simulink model "Electromech_sys_current_lin_obs"  (R2025b)
settings: Solver=VariableStepAuto  StartTime=0.0  StopTime=10.0  RelTol=1e-3
values from neighbouring files (symbols this model uses):
  A = (J - R) * Hxx    [linearize_electromech.m]    (also in linearize_mech.m = (J - R) * Hxx + grad_g * u_eq_mech)
  B = g    [linearize_electromech.m]    (also in linearize_mech.m)
  i_eq = - (1/re) * dHdQ_eq + (1/re) * u_op    [equilibrium_electromech.m]
  p_0 = 0    [Init_Simulink_param_lin_Electromech.m]
  ptilde_0 = phat_0 - x_eq(2)    [Init_Simulink_param_lin_Electromech.m]
  q_0 = 0    [Init_Simulink_param_lin_Electromech.m]
  Q_0 = 0    [Init_Simulink_param_lin_Electromech.m]
  qtilde_0 = qhat_0 - x_eq(1)    [Init_Simulink_param_lin_Electromech.m]
  Qtilde_0 = Qhat_0 - x_eq(3)    [Init_Simulink_param_lin_Electromech.m]
  x_eq = [q_eq; p_eq; Q_eq]    [equilibrium_electromech.m]
undefined symbols (not defined in the file or in its folder): Cnum, params, u_eq
settings Model: Creator=filippougolini  LastModifiedBy=filippougolini

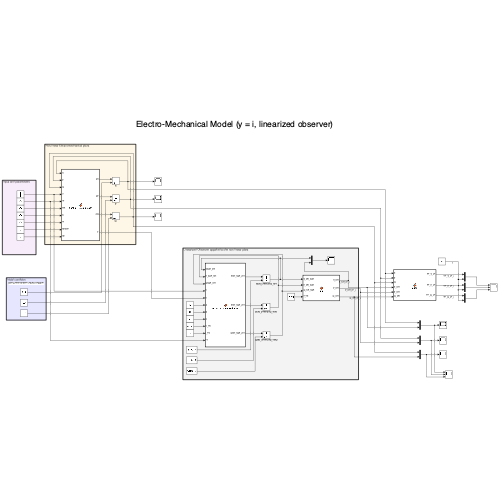
[thumbnail: Simulink's stored preview of the top-level diagram]
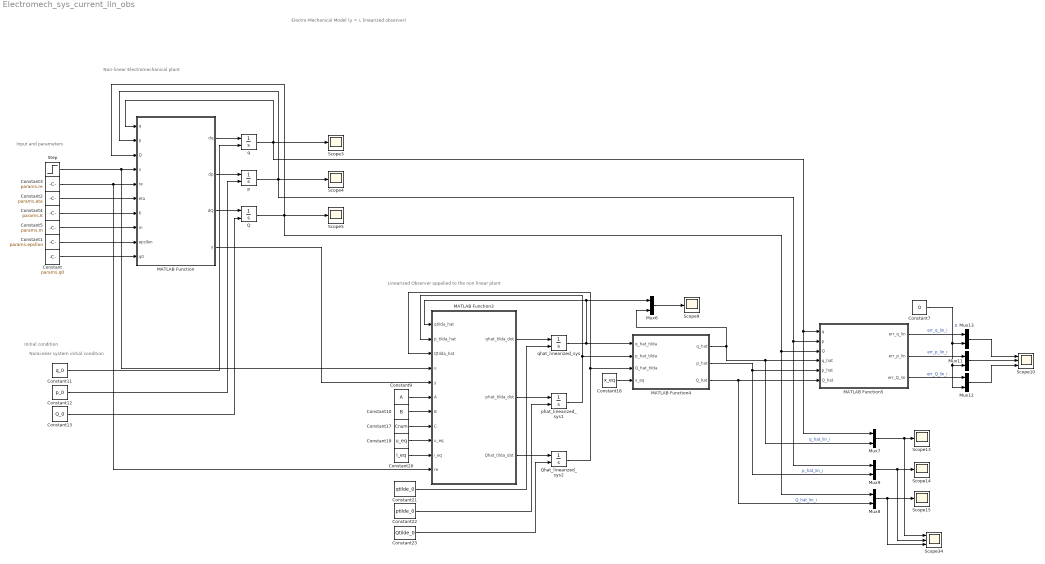
== system Electromech_sys_current_lin_obs ==
  note: Linearized Observer appalied to the non linear plant
  note: Input and parameters
  note: NonLinear system initial condition
  note: Non-linear Electromechanical plant
  note: Electro-Mechanical Model (y = i, linearized observer)
  note: Initial condition
  Constant : Constant  Value=params.q0
  Constant1 : Constant  Value=params.epsllon
  Constant10 : Constant  Value=B
  Constant11 : Constant  Value=q_0
  Constant12 : Constant  Value=p_0
  Constant13 : Constant  Value=Q_0
  Constant17 : Constant  Value=Cnum
  Constant18 : Constant  Value=x_eq
  Constant19 : Constant  Value=u_eq
  Constant2 : Constant  Value=params.eta
  Constant20 : Constant  Value=i_eq
  Constant21 : Constant  Value=qtilde_0
  Constant22 : Constant  Value=ptilde_0
  Constant23 : Constant  Value=Qtilde_0
  Constant3 : Constant  Value=params.re
  Constant4 : Constant  Value=params.K
  Constant5 : Constant  Value=params.m
  Constant7 : Constant  Value=0
  Constant9 : Constant  Value=A
  MATLAB Function : MATLAB Function  TreatAsAtomicUnit=on
  MATLAB Function3 : MATLAB Function  TreatAsAtomicUnit=on
  MATLAB Function4 : MATLAB Function  TreatAsAtomicUnit=on
  MATLAB Function5 : MATLAB Function  TreatAsAtomicUnit=on
  Mux{6..9,11..13} (7 alike) : Mux  Inputs=2
  Q : Integrator  InitialConditionSource=external
  Qhat_linearized_sys2 : Integrator  InitialConditionSource=external  InitialCondition=20e-5
  Scope10 : Scope  NumInputPorts=3
      settings: ActiveDisplayString=3  ActiveDisplayYMinimum=-9.7438576334412446E-8  ActiveDisplayYMaximum=3.7694718700971209E-7  DataLoggingVariableName=ScopeData10
  Scope{3..5,9,13..15} (7 alike) : Scope
      Scope13 settings: ActiveDisplayYMinimum=-0.00014562196235781276  ActiveDisplayYMaximum=0.0013105976612203152  DataLoggingVariableName=ScopeData13
      Scope14 settings: ActiveDisplayYMinimum=-0.0045902088543352884  ActiveDisplayYMaximum=0.00516486271210546  DataLoggingVariableName=ScopeData14
      Scope15 settings: ActiveDisplayYMinimum=-2.096197823231283E-8  ActiveDisplayYMaximum=1.8865780409081551E-7  DataLoggingVariableName=ScopeData15
      Scope3 settings: ActiveDisplayYMinimum=-4.0944874698701246E-5  ActiveDisplayYMaximum=0.0003685038722883113  DataLoggingVariableName=ScopeData3
      Scope4 settings: ActiveDisplayYMinimum=-1  ActiveDisplayYMaximum=1  DataLoggingVariableName=ScopeData4
      Scope5 settings: ActiveDisplayYMinimum=-1  ActiveDisplayYMaximum=1  DataLoggingVariableName=ScopeData5
      Scope9 settings: ActiveDisplayYMinimum=-0.0028704641819507128  ActiveDisplayYMaximum=0.00068289488649407159  DataLoggingVariableName=ScopeData9
  Scope34 : Scope  NumInputPorts=3
      settings: ActiveDisplayString=3  ActiveDisplayYMinimum=-3.7694718700971209E-7  ActiveDisplayYMaximum=9.7438576334412446E-8  DataLoggingVariableName=ScopeData34
  Step : Step  After=5e3  SampleTime=0
  p : Integrator  InitialConditionSource=external
  phat_linearized_sys1 : Integrator  InitialConditionSource=external  InitialCondition=20e-5
  q : Integrator  InitialConditionSource=external
  qhat_linearized_sys : Integrator  InitialConditionSource=external  InitialCondition=20e-5
  wires:
  Constant5/1 -> MATLAB Function/8(m)
  Mux13/1 -> Scope10/1
  Constant13/1 -> Q/2
  qhat_linearized_sys/1 -> MATLAB Function3/1(qtilda_hat), Mux6/1, MATLAB Function4/1(q_hat_tilda)
  Constant17/1 -> MATLAB Function3/8(C)
  MATLAB Function3/1(qhat_tilda_dot) -> qhat_linearized_sys/1
  Constant9/1 -> MATLAB Function3/6(A)
  Mux9/1 -> Scope34/2, Scope14/1
  Step/1 -> MATLAB Function3/4(u), MATLAB Function/4(u)
  Constant12/1 -> p/2
  Constant19/1 -> MATLAB Function3/9(u_eq)
  Constant20/1 -> MATLAB Function3/10(i_eq)
  Qhat_linearized_sys2/1 -> MATLAB Function3/3(Qtilda_hat), MATLAB Function4/3(Q_hat_tilda)
  Mux7/1 -> Scope34/1, Scope13/1
  MATLAB Function4/2(p_hat) -> MATLAB Function5/5(p_hat), Mux9/2  "p_hat_lin_i"
  Constant10/1 -> MATLAB Function3/7(B)
  p/1 -> MATLAB Function5/2(p), Mux9/1, MATLAB Function/2(p), Scope4/1
  Constant3/1 -> MATLAB Function3/11(re), MATLAB Function/5(re)
  Constant23/1 -> Qhat_linearized_sys2/2
  Constant1/1 -> MATLAB Function/9(epsllon)
  Constant/1 -> MATLAB Function/10(q0)
  phat_linearized_sys1/1 -> MATLAB Function3/2(p_tilda_hat), MATLAB Function4/2(p_hat_tilda)
  q/1 -> MATLAB Function5/1(q), Mux7/1, Scope3/1, MATLAB Function/1(q)
  Mux6/1 -> Scope9/1
  MATLAB Function5/3(err_Q_lin) -> Mux12/1  "err_Q_lin_i"
  MATLAB Function4/3(Q_hat) -> MATLAB Function5/6(Q_hat), Mux8/2  "Q_hat_lin_i"
  Constant7/1 -> Mux12/2, Mux11/2, Mux13/2  "0"
  MATLAB Function/3(dQ) -> Q/1
  MATLAB Function/1(dq) -> q/1
  MATLAB Function5/2(err_p_lin) -> Mux11/1  "err_p_lin_i"
  MATLAB Function/2(dp) -> p/1
  MATLAB Function/4(y) -> MATLAB Function3/5(y)
  Q/1 -> MATLAB Function5/3(Q), Mux8/1, MATLAB Function/3(Q), Scope5/1
  MATLAB Function5/1(err_q_lin) -> Mux13/1  "err_q_lin_i"
  Constant2/1 -> MATLAB Function/6(eta)
  Constant21/1 -> qhat_linearized_sys/2
  Constant4/1 -> MATLAB Function/7(K)
  Mux11/1 -> Scope10/2
  MATLAB Function3/3(Qhat_tilda_dot) -> Qhat_linearized_sys2/1
  Constant18/1 -> MATLAB Function4/4(x_eq)
  Constant22/1 -> phat_linearized_sys1/2
  Mux8/1 -> Scope34/3, Scope15/1
  Mux12/1 -> Scope10/3
  MATLAB Function3/2(phat_tilda_dot) -> phat_linearized_sys1/1
  Constant11/1 -> q/2
  MATLAB Function4/1(q_hat) -> Mux6/2, MATLAB Function5/4(q_hat), Mux7/2  "q_hat_lin_i"

== matlab function Electromech_sys_current_lin_obs/MATLAB Function4 ==
  data: q_hat_tilda input; p_hat_tilda input; Q_hat_tilda input; x_eq input; q_hat output; p_hat output; Q_hat output
function [q_hat, p_hat, Q_hat] = fcn(q_hat_tilda, p_hat_tilda, Q_hat_tilda, ...
    x_eq)
    
    q_tilda_eq = x_eq(1);
    p_tilda_eq = x_eq(2);
    Q_tilda_eq = x_eq(3);

    
    
    q_hat = q_hat_tilda + q_tilda_eq;
    p_hat = p_hat_tilda + p_tilda_eq;
    Q_hat = Q_hat_tilda + Q_tilda_eq;
end

== matlab function Electromech_sys_current_lin_obs/MATLAB Function5 ==
  data: q input; err_q_lin output; p input; Q input; q_hat input; p_hat input; Q_hat input; err_p_lin output; err_Q_lin output
function [err_q_lin, err_p_lin, err_Q_lin] = error(q, p, Q, q_hat, p_hat, Q_hat)

    err_q_lin = q - q_hat;
    err_p_lin = p - p_hat;
    err_Q_lin = Q - Q_hat;
end

== matlab function Electromech_sys_current_lin_obs/MATLAB Function ==
  data: q input; p input; Q input; u input; dq output; re input; eta input; K input; m input; epsllon input; q0 input; dp output; dQ output; y output
function [dq, dp, dQ, y] = plant_pH_electromech(q, p, Q, u, re, eta, K, m, epsllon, q0)
% Electro-mechanical pH plant

    % Parameters: m, K, eta, eps, re, q0 in workspace

    J = [  0  1  0;
          -1  0  0;
           0  0  0 ];

    R = diag([0, eta, 1/re]);
    g = [0; 0; 1/re];

    % Hamiltonian gradient gradH(q,p,Q)
    Cq   = epsllon * (q + q0)^4;

    dHdq = K*q - 2*Q^2 / (epsllon * (q + q0)^5);
    dHdp = p / m;
    dHdQ = Q / Cq;

    gradH = [dHdq; dHdp; dHdQ];

    xdot = (J - R) * gradH + g*u;

    y = - (1/re) * dHdQ + (1/re) * u; % i = Q_dot
    
    dq = xdot(1);
    dp = xdot(2);
    dQ = xdot(3);
end

== matlab function Electromech_sys_current_lin_obs/MATLAB Function3 ==
  data: qhat_tilda_dot output; phat_tilda_dot output; Qhat_tilda_dot output; qtilda_hat input; p_tilda_hat input; Qtilda_hat input; u input; y input; A input; B input; C input; u_eq input; i_eq input; re input
function [qhat_tilda_dot, phat_tilda_dot, Qhat_tilda_dot] = ...
    observer_linearized_dev(qtilda_hat, p_tilda_hat, Qtilda_hat, u, y, A, ...
    B, C, u_eq, i_eq, re)

    % ---- Deviation state and absolute estimate ---- 
    delta_xhat = [qtilda_hat; p_tilda_hat; Qtilda_hat]; % 3x1 
    % ---- Deviation input and output ---- 
    delta_u = u - u_eq; 
    delta_y = y - i_eq;
    
    g = [0; 0; 1/re];
    gamma = 20;
    L  = gamma * g;
    
    delta_xhatdot = A*delta_xhat + B*delta_u + L' * (delta_y - C'*delta_xhat);
    

    % ---- Derivatives of deviation states ---- 
    qhat_tilda_dot = delta_xhatdot(1); 
    phat_tilda_dot = delta_xhatdot(2); 
    Qhat_tilda_dot = delta_xhatdot(3);
end
